simulink model "ltc2607_task"  (Simulink 3.00)
libraries: mathlib x5, speclib x1, genlib x1

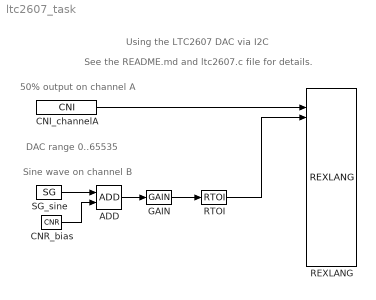
== system ltc2607_task ==
  note: Using the LTC2607 DAC via I2C
  note: See the README.md and ltc2607.c file for details.
  note: 50% output on channel A
  note: DAC range 0..65535
  note: Sine wave on channel B
  ADD : mathlib/ADD
  CNI_channelA : mathlib/CNI  icn=32768
  CNR_bias : mathlib/CNR  ycn=0.5
  GAIN : mathlib/GAIN  k=65535
  REXLANG : speclib/REXLANG  SystemSampleTime=-1  tab_matlab=BASIC  srcname=ltc2607.c  srctype=1: STL  stack=0  debug=1: No check  p0=0  p1=0  p2=0  p3=0  p4=0  p5=0  p6=0  p7=0  p8=0  p9=0  p10=0  p11=0  p12=0  p13=0  p14=0  p15=0  fname=/dev/i2c-1
  RTOI : mathlib/RTOI
  SG_sine : genlib/SG  isig=1: SINE  amp=0.5  freq=0.1  phase=0  ifrunit=1: Hz  iphunit=1: degrees
  wires:
  CNI_channelA/1 -> REXLANG/2
  ADD/1 -> GAIN/1
  CNR_bias/1 -> ADD/2
  GAIN/1 -> RTOI/1
  RTOI/1 -> REXLANG/3
  SG_sine/1 -> ADD/1
